simulink model "Motor_Test_All"  (R2015b)
settings: Solver=FixedStepAuto  StartTime=0.0  StopTime=100.0  RelTol=1e-3
undefined symbols (not defined in the file): sigbuilder_block
libraries: simulink x1
settings Model: SimulationMode=external  ExtModeTrigDuration=2  Creator=Joern  LastModifiedBy=Joern
settings OptimizationCC: OptimizeModelRefInitCode=on  LifeSpan=1  MaxStackSize=64
settings HardwareCC: ProdBitPerInt=16  ProdBitPerPointer=16  ProdLargestAtomicFloat=None  ProdWordSize=8  ProdHWDeviceType=Atmel->AVR
settings ModelReferenceCC: ParallelModelReferenceMATLABWorkerInit=Load Top Model
settings RTWCC: SystemTargetFile=ert.tlc  TemplateMakefile=ert_default_tmf  Description=Embedded Coder  Toolchain=Arduino AVR v1.6.1  BuildConfiguration=Faster Runs
settings CodeAppCC: IgnoreCustomStorageClasses=off
settings ERTTargetCC: GenerateSampleERTMain=on  SupportContinuousTime=on  SupportVariableSizeSignals=on

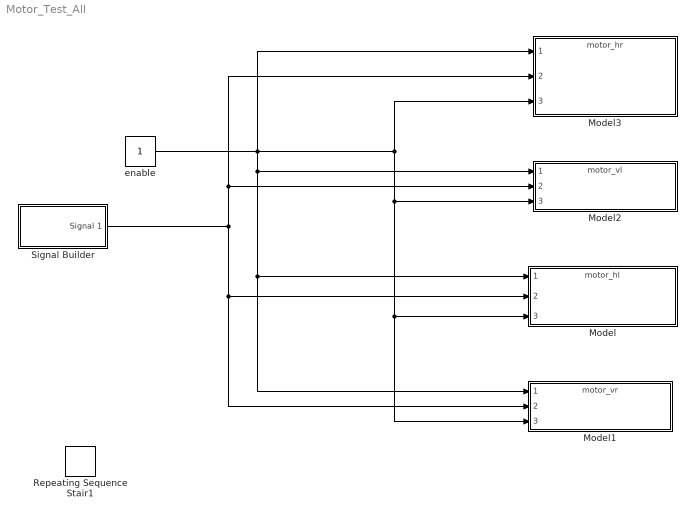
== system Motor_Test_All ==
  Model : ModelReference  ModelNameDialog=motor_hl.slx  SimulationMode=Normal  ModelReferenceVersion=1.4  CopyOfModelName=motor_hl.slx
  Model1 : ModelReference  ModelNameDialog=motor_vr.slx  SimulationMode=Normal  ModelReferenceVersion=1.4  CopyOfModelName=motor_vr.slx
  Model2 : ModelReference  ModelNameDialog=motor_vl.slx  SimulationMode=Normal  ModelReferenceVersion=1.4  CopyOfModelName=motor_vl.slx
  Model3 : ModelReference  ModelNameDialog=motor_hr.slx  SimulationMode=Normal  ModelReferenceVersion=1.6  CopyOfModelName=motor_hr.slx
  Repeating Sequence Stair1 : simulink/Sources/Repeating Sequence Stair  OutValues=[0 50 100 150 200 255 200 150 100 50 0 0 0 0 0 0 0 0].'  tsamp=10  OutMin=[]  OutMax=[]  OutDataTypeStr=double  OutputDataTypeScalingMode=double  OutDataType=fixdt(0,8)  ConRadixGroup=Best Precision: Vector-wise  OutScaling=2^-12
  Signal Builder : Subsystem  Tag=STV Subsys  LoadFcn=sigbuilder_block('load');  StartFcn=sigbuilder_block('start');  StopFcn=sigbuilder_block('stop');  ClipboardFcn=sigbuilder_block('clipboard');  mask(Sigbuilder block){}
      mask help: Simulink:masks:SigbuilderBlock_MD
      mask init:
      | if ~strcmp(get_param(bdroot(gcbh),'SimulationStatus'),'stopped') tuvar = sigbuilder_block('maskInit'); end
      settings: CopyFcn=sigbuilder_block('copy');  DeleteFcn=sigbuilder_block('delete');  ModelCloseFcn=sigbuilder_block('modelClose');  PreSaveFcn=sigbuilder_block('preSave');  PauseFcn=sigbuilder_block('pause');  ContinueFcn=sigbuilder_block('continue');  NameChangeFcn=sigbuilder_block('namechange');  OpenFcn=sigbuilder_block('open',[6 30 1012.5 447.75 ]);  CloseFcn=sigbuilder_block('close');
      mask Display: plot(0, 0, 100, 100,[2, 2, 32, 32, 2], [68, 8, 8, 68, 68],[32, 2], [38, 38], [32, 19, 2],[53, 60, 44], [32, 17, 17, 2],[16, 16, 31, 31]);txt = getActiveGroup(gcbh);text(2, 100, txt,'verticalAlignment', 'top');
  enable : Constant
  wires:
  Signal Builder/1(Signal 1) -> Model2/2, Model3/2, Model1/2, Model/2
  enable/1 -> Model1/3, Model/3, Model2/3, Model3/3, Model3/1, Model1/1, Model/1, Model2/1

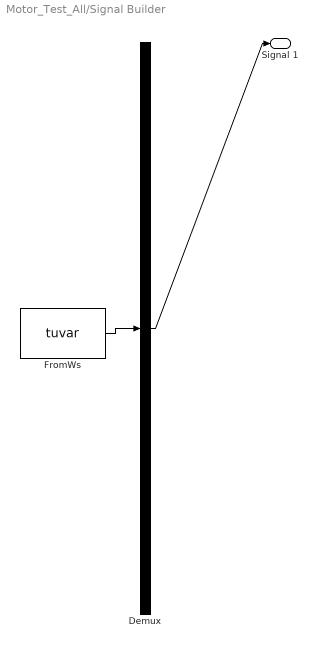
== system Motor_Test_All/Signal Builder ==
  Demux : Demux  Tag=STV Demux  Outputs=1
  FromWs : FromWorkspace  Tag=STV FromWs  VariableName=tuvar  SampleTime=0
      SigBuilderData=|
      | common.afterFinalStr = 'Extrapolate'
      | common.sampleTime = 0
      | dataSet.timeRange = [0 7]
      | dataSet.name = 'Group 1'
      | sbobj.Groups.Name = 'Group 1'
      | sbobj.Groups.Signals.Name = 'Signal 1'
      | sbobj.Groups.Signals.XData = [0 1 2 4 6 7]
      | sbobj.Groups.Signals.YData = [0 128 128 255 255 0]
      | sbobj.Groups.TimeRange = [0 7]
  Signal 1 : Outport  Tag=STV Outport
  wires:
  FromWs/1 -> Demux/1
  Demux/1 -> Signal 1/1
